simulink model "MultiUAV_DroneShow"  (R2026a)
settings: Solver=ode1  StopTime=74.3333  FixedStep=Ts_sim  MaxStep=0.01  AbsTol=1e-6
PreLoadFcn:
  | setupParams
values from neighbouring files (symbols this model uses):
  arm_duration = 2    [setupParams.m]
  gnss_deny_mask = false(N_uav, 1)    [setupParams.m]
  gnss_err_gain = sqrt(1 - gnss_err_pole^2)    [setupParams.m]
  gnss_err_pole = exp(-Ts_sim / gnss_err_tau)    [setupParams.m]
  gnss_err_seed = reshape(40000 + (1:(N_uav * 3)), N_uav, 3)    [setupParams.m]
  gps_accuracy_rtk_fix = 0.02    [setupParams.m]
  gps_lock_duration = 2    [setupParams.m]
  gravity = 9.81    [setupParams.m]
  hb_period_ticks = mavlink_hb_interval / Ts_sim    (= 100)    [setupParams.m]
  init_positions = init_positions(pad_of, :)    [planShow.m]    (also in setupParams.m = plan.init_positions)
  Kd_pos = repmat([Kd_xy Kd_xy Kd_z], N_uav, 1)    [setupParams.m]
  Kff_pos = Kd_pos    [setupParams.m]
  Kp_pos = repmat([Kp_xy Kp_xy Kp_z], N_uav, 1)    [setupParams.m]
  land_end_time = plan.land_end_time    [packShowUpload.m]    (also in planShow.m = show_flight_duration + land_duration; setupParams.m)
  land_speed = cfg.land_speed    [planShow.m]
  land_start_time = show_flight_duration    [planShow.m]    (also in setupParams.m = plan.land_start_time)
  land_total_duration = land_duration + land_settle    [planShow.m]    (also in setupParams.m = plan.land_total_duration)
  mav_sys_span = 250    [setupParams.m]
  N_uav = 20    [DroneShowExample.m]    (also in packShowUpload.m = cfg.N_uav; planShow.m = cfg.N_uav; setupParams.m = 10)
  num_waypoints = length(upload_times)    [packShowUpload.m]    (also in setupParams.m = pack.num_waypoints)
  rtcm_data_bytes = 180    [setupParams.m]
  rtcm_interval = 1.0    (= 1)    [setupParams.m]
  rtcm_payload_bytes = 4 * 4 * rtk_n_sat    [setupParams.m]
  rtcm_period_ticks = rtcm_interval / Ts_sim    (= 100)    [setupParams.m]
  rtk_amb_l1_base = 1000000 + mod(97 * (1:rtk_n_sat)', 1009)    [setupParams.m]
  rtk_amb_l1_rover = rtk_amb_l1_base + rtk_amb_l1    [setupParams.m]
  rtk_amb_l2_base = 1000000 + mod(89 * (1:rtk_n_sat)', 1009)    [setupParams.m]
  rtk_amb_l2_rover = rtk_amb_l2_base + rtk_amb_l2    [setupParams.m]
  rtk_base_lla = [42.3601, -71.0589, 10]    [setupParams.m]
  rtk_deny_mask = false(N_uav, 1)    [setupParams.m]
  rtk_f1 = 1575.42e6    (= 1575420000)    [setupParams.m]
  rtk_f2 = 1227.60e6    (= 1227600000)    [setupParams.m]
  rtk_fall_slew = -gps_accuracy_standard / reconverge_time    (= -0.3)    [setupParams.m]
  rtk_fix_thresh_l1 = 0.30    (= 0.3)    [setupParams.m]
  rtk_fix_thresh_wl = 0.25    [setupParams.m]
  rtk_inject_enable = double(~skip_preflight | rtk_deny_mask(:)')    [setupParams.m]
  rtk_lambda1 = rtk_c / rtk_f1    (= 0.190293672798)    [setupParams.m]
  rtk_lambda2 = rtk_c / rtk_f2    (= 0.244210213425)    [setupParams.m]
  rtk_lambda_wl = rtk_c / (rtk_f1 - rtk_f2)    (= 0.861918400322)    [setupParams.m]
  rtk_lock_dwell = 2.0    (= 2)    [setupParams.m]
  rtk_los = [cosd(rtk_el) .* sind(rtk_az), cosd(rtk_el) .* cosd(rtk_az), sind(rtk_el)]    [setupParams.m]
  rtk_mean_clk = zeros(2, 1)    [setupParams.m]
  rtk_mean_obs = zeros(2, rtk_n_sat)    [setupParams.m]
  rtk_n_sat = numel(rtk_az)    [setupParams.m]
  rtk_rough_range = pseudoranges(rtk_base_lla, rtk_sat_pos, 'RangeAccuracy', 0)    [setupParams.m]
  rtk_sat_pos = rtk_sat_pos_all(rtk_vis, :)    [setupParams.m]
  rtk_seedm_clk = 9101 + 8 * rtk_n_sat + (0:1)'    [setupParams.m]
  rtk_seedm_l1 = rtk_seedm_p2 + 2 * rtk_n_sat    [setupParams.m]
  rtk_seedm_l2 = rtk_seedm_l1 + 2 * rtk_n_sat    [setupParams.m]
  rtk_seedm_p1 = 9101 + reshape(0:2 * rtk_n_sat - 1, 2, rtk_n_sat)    [setupParams.m]
  rtk_seedm_p2 = rtk_seedm_p1 + 2 * rtk_n_sat    [setupParams.m]
  rtk_sigma_bp = [0, rtk_timeout, rtk_float_timeout]    [setupParams.m]
  rtk_sigma_table = sqrt(max(0, rtk_sigma_tiers.^2 - gps_accuracy_rtk_fix^2))    [setupParams.m]
  rtk_sigma_unfixed = 0.75    [setupParams.m]
  rtk_slip_thresh_l1 = 0.02    [setupParams.m]
  rtk_slip_thresh_wl = 0.10    (= 0.1)    [setupParams.m]
  rtk_status_l1 = 1    [setupParams.m]
  rtk_status_unfixed = 3    [setupParams.m]
  rtk_timeout = 2.5    [setupParams.m]
  rtk_var_clk = rtk_clock_sigma^2 * ones(2, 1)    [setupParams.m]
  rtk_var_l = [rtk_sigma_phase_base^2; rtk_sigma_phase_rover^2] * ones(1, rtk_n_sat)    [setupParams.m]
  rtk_var_p = [rtk_sigma_code_base^2;  rtk_sigma_code_rover^2 ] * ones(1, rtk_n_sat)    [setupParams.m]
  skip_preflight = traj_source == 1    [DroneShowExample.m]    (also in setupParams.m = false)
  st_period_ticks = mavlink_st_interval / Ts_sim    (= 100)    [setupParams.m]
  st_phase_ticks = st_period_ticks / 2    (= 50)    [setupParams.m]
  telemetry_tx_enable = double(~skip_preflight)    [setupParams.m]
  traj_upload_flat = zeros(N_uav*num_waypoints, 7)    [packShowUpload.m]    (also in setupParams.m = pack.traj_upload_flat)
  Ts_sim = cfg.Ts_sim    [packShowUpload.m]    (also in setupParams.m = 0.01)
  uav_loss_seed = 31000 + (1:N_uav)    [setupParams.m]
  uav_mass = 0.1    [setupParams.m]
  upload_duration = (total_packets + N_uav) * Ts_sim * 1.2    [packShowUpload.m]    (also in setupParams.m = pack.upload_duration)
  upload_rate_vec = [1 ./ upload_dt; 1 / upload_dt(end)]    [packShowUpload.m]    (also in setupParams.m = pack.upload_rate_vec)
  upload_request = traj_source == 2    [DroneShowExample.m]
undefined symbols (not defined in the file or in its folder): abort_request, DiscIntNeverNeededParam, doppler, loss_seed, packet_loss_rate, Payload, SystemID, uav_loss_rate
libraries: uavmavlinklib x22, hdlsllib x16, dspsigops x8, simulink x7, matrix_library x4, commchan3 x2, etargetslib x1, uavalgslib x1, sensorinslib x1, slpidlib x1, dspmathops x1, commrandsrc3 x1
(part 3 of 4)

== system MultiUAV_DroneShow/BaseStation/Transmitter/MissionItemTx/AddrSplit ==
  idx : Inport
  AddC1 : Sum  OutDataTypeStr=uint16
  AddS1 : Sum  OutDataTypeStr=uint16
  C_one : Constant  Value=uint16(1)  OutDataTypeStr=uint16
  C_span : Constant  Value=uint16(mav_sys_span)  OutDataTypeStr=uint16
  C_zero : Constant  Value=uint8(0)  OutDataTypeStr=uint8
  DTC_comp : DataTypeConversion  OutDataTypeStr=uint8
  DTC_sys : DataTypeConversion  OutDataTypeStr=uint8
  DivF : Product  Inputs=*/  OutDataTypeStr=uint16
  MaxIdx : MinMax  Function=max  Inputs=2  OutDataTypeStr=uint16
  MulS : Product  Inputs=**  OutDataTypeStr=uint16
  Sub1 : Sum  Inputs=+-  OutDataTypeStr=uint16
  SubS : Sum  Inputs=+-  OutDataTypeStr=uint16
  SwComp : Switch  Criteria=u2 > Threshold
  SwSys : Switch  Criteria=u2 > Threshold
  target_system : Outport
  target_component : Outport  Port=2
  wires:
  idx/1 -> MaxIdx/1, SwSys/2, SwComp/2
  C_one/1 -> MaxIdx/2, Sub1/2, AddS1/2, AddC1/2
  MaxIdx/1 -> Sub1/1
  Sub1/1 -> DivF/1, SubS/1
  C_span/1 -> DivF/2, MulS/2
  DivF/1 -> MulS/1, AddC1/1
  MulS/1 -> SubS/2
  SubS/1 -> AddS1/1
  AddS1/1 -> DTC_sys/1
  AddC1/1 -> DTC_comp/1
  DTC_sys/1 -> SwSys/1
  C_zero/1 -> SwSys/3, SwComp/3
  DTC_comp/1 -> SwComp/1
  SwSys/1 -> target_system/1
  SwComp/1 -> target_component/1

== system MultiUAV_DroneShow/BaseStation/Transmitter/RTCMTx/PackRTKDataBlk ==
  BaseObs : Inport
  BytePack : etargetslib/Byte Pack  datatypes={'single'}  byteAlign=1
  ConcatBytes : Concatenate
  DTC_single : DataTypeConversion  OutDataTypeStr=single
  PadZeros : Constant  Value=zeros(1,rtcm_data_bytes-rtcm_payload_bytes,'uint8')  OutDataTypeStr=uint8
  data : Outport
  wires:
  BytePack/1 -> ConcatBytes/1
  ConcatBytes/1 -> data/1
  PadZeros/1 -> ConcatBytes/2
  BaseObs/1 -> DTC_single/1
  DTC_single/1 -> BytePack/1

== system MultiUAV_DroneShow/DroneFleet/SetpointGenerator/PlannedTrajectory/OnboardTrajSource ==
  ShowTime : Inport
  BufferAsWpDroneXYZ : Reshape  OutputDimensionality=Customize  OutputDimensions=[num_waypoints, N_uav, 3]
  CatPosVelYaw : Concatenate  NumInputs=3  Mode=Multidimensional array  ConcatenateDimension=2
  FracOfDelta : Product
  GroundHold : Constant  Value=[init_positions'; zeros(4, N_uav)]
  IdxNext : Bias  Bias=2
  IdxThis : Bias  Bias=1
  NextWpPerDrone : Reshape  OutputDimensionality=Customize  OutputDimensions=[N_uav 3]
  OnboardPos : Sum  Inputs=|++
  OnboardVel : Product
  OnboardYaw : Constant  Value=zeros(N_uav,1)
  PickNextWp : Selector  NumberOfDimensions=3  IndexOptions=Index vector (port),Select all,Select all  Indices=1,1,1  OutputSizes=1,1,1
  PickThisWp : Selector  NumberOfDimensions=3  IndexOptions=Index vector (port),Select all,Select all  Indices=1,1,1  OutputSizes=1,1,1
  PickWpRate : Selector  InputPortWidth=num_waypoints  IndexOptions=Index vector (port)  Indices=1  OutputSizes=1
  PreShowGate : Switch  Criteria=u2 > Threshold
  ReadOnboardBuffer : DataStoreRead  DataStoreName=OnboardBuffer  IndexOptions=Index vector (dialog)  Indices=1  OutputSizes=1
  ThisWpPerDrone : Reshape  OutputDimensionality=Customize  OutputDimensions=[N_uav 3]
  ToSevenRows : Math  Operator=transpose
  WaypointLookup : PreLookup  BreakpointsData=upload_times
  WpDelta : Sum  Inputs=+-
  WpRateVec : Constant  Value=upload_rate_vec
  TrajMatrix : Outport
  wires:
  ShowTime/1 -> WaypointLookup/1, PreShowGate/2  "show_time"
  PickWpRate/1 -> OnboardVel/2
  WpRateVec/1 -> PickWpRate/1
  OnboardVel/1 -> CatPosVelYaw/2
  PreShowGate/1 -> TrajMatrix/1  "onboard_traj"
  GroundHold/1 -> PreShowGate/3
  ToSevenRows/1 -> PreShowGate/1
  CatPosVelYaw/1 -> ToSevenRows/1
  OnboardYaw/1 -> CatPosVelYaw/3
  OnboardPos/1 -> CatPosVelYaw/1  "onboard_pos"
  FracOfDelta/1 -> OnboardPos/2
  WpDelta/1 -> OnboardVel/1, FracOfDelta/2  "wp_delta"
  WaypointLookup/2 -> FracOfDelta/1
  ThisWpPerDrone/1 -> OnboardPos/1, WpDelta/2
  NextWpPerDrone/1 -> WpDelta/1
  PickNextWp/1 -> NextWpPerDrone/1
  PickThisWp/1 -> ThisWpPerDrone/1
  IdxNext/1 -> PickNextWp/2
  IdxThis/1 -> PickWpRate/2, PickThisWp/2
  BufferAsWpDroneXYZ/1 -> PickNextWp/1, PickThisWp/1
  ReadOnboardBuffer/1 -> BufferAsWpDroneXYZ/1  "onboard_wp"
  WaypointLookup/1 -> IdxNext/1, IdxThis/1

== system MultiUAV_DroneShow/DroneFleet/Transmitter/MissionAckEncoder/AckMsgGate ==
  In1 : Inport
  Enable : EnablePort
  AckType0 : Constant  Value=uint8(0)  OutDataTypeStr=uint8
  AddrSplit : Subsystem
  BlankMsg_MAck : uavmavlinklib/MAVLink Blank Message  dialectSource=Select from standard MAVLink dialects  dialect=common.xml  dialectCustom=common.xml  version=2  messageType=MISSION_ACK  SystemID=1  ComponentID=1  SampleTime=inf
  DTC_MAck : DataTypeConversion  OutDataTypeStr=uint8  SaturateOnIntegerOverflow=off  RndMeth=Floor
  Fill_MAck : BusAssignment  AssignedSignals=Payload.target_system,Payload.type,Payload.target_component
  Pad_MAck : dspsigops/Pad  padAlong=Rows  dimsToPad=1  valSrc=Specify via dialog  padVal=0  spec=Output size  padNumOutRowsSpecMethod=User-specified  numOutRows=1  padNumOutColsSpecMethod=User-specified  numOutCols=40  isVarDimsMode=off  padBeginning=0  padEnd=0  outSizeMode=User-specified  outSize=1  padSigAt=End  trunc_flag=None  roundingMode=Floor  overflowMode=off  truncOrWrapMode=Truncate  wrap_flag=None
  Ser_MAck : uavmavlinklib/MAVLink Serializer  dialectSource=Select from standard MAVLink dialects  dialect=common.xml  dialectCustom=common.xml  version=2  messageType=MISSION_ACK
  TermSerMAckLen : Terminator
  Out1 : Outport
  wires:
  Ser_MAck/1 -> Pad_MAck/1
  Ser_MAck/2 -> TermSerMAckLen/1
  BlankMsg_MAck/1 -> Fill_MAck/1
  Pad_MAck/1 -> DTC_MAck/1
  AckType0/1 -> Fill_MAck/3
  DTC_MAck/1 -> Out1/1
  Fill_MAck/1 -> Ser_MAck/1
  In1/1 -> AddrSplit/1(idx)
  AddrSplit/1(target_system) -> Fill_MAck/2
  AddrSplit/2(target_component) -> Fill_MAck/4

== system MultiUAV_DroneShow/DroneFleet/Transmitter/MissionRequestEncoder/ReqMsgGate ==
  In1 : Inport
  In2 : Inport  Port=2
  Enable : EnablePort
  AddrSplit : Subsystem
  BlankMsg_MReq : uavmavlinklib/MAVLink Blank Message  dialectSource=Select from standard MAVLink dialects  dialect=common.xml  dialectCustom=common.xml  version=2  messageType=MISSION_REQUEST_INT  SystemID=1  ComponentID=1  SampleTime=inf
  DTC_MReq : DataTypeConversion  OutDataTypeStr=uint8  SaturateOnIntegerOverflow=off  RndMeth=Floor
  Fill_MReq : BusAssignment  AssignedSignals=Payload.target_system,Payload.seq,Payload.target_component
  Pad_MReq : dspsigops/Pad  padAlong=Rows  dimsToPad=1  valSrc=Specify via dialog  padVal=0  spec=Output size  padNumOutRowsSpecMethod=User-specified  numOutRows=1  padNumOutColsSpecMethod=User-specified  numOutCols=40  isVarDimsMode=off  padBeginning=0  padEnd=0  outSizeMode=User-specified  outSize=1  padSigAt=End  trunc_flag=None  roundingMode=Floor  overflowMode=off  truncOrWrapMode=Truncate  wrap_flag=None
  Ser_MReq : uavmavlinklib/MAVLink Serializer  dialectSource=Select from standard MAVLink dialects  dialect=common.xml  dialectCustom=common.xml  version=2  messageType=MISSION_REQUEST_INT
  TermSerMReqLen : Terminator
  Out1 : Outport
  wires:
  BlankMsg_MReq/1 -> Fill_MReq/1
  Fill_MReq/1 -> Ser_MReq/1
  Ser_MReq/2 -> TermSerMReqLen/1
  Pad_MReq/1 -> DTC_MReq/1
  Ser_MReq/1 -> Pad_MReq/1
  In2/1 -> Fill_MReq/3
  DTC_MReq/1 -> Out1/1
  In1/1 -> AddrSplit/1(idx)
  AddrSplit/1(target_system) -> Fill_MReq/2
  AddrSplit/2(target_component) -> Fill_MReq/4

== system MultiUAV_DroneShow/RTKBase/ObservableSource/Simulated/ObservableGen ==
  RoverPos : Inport
  BreakLoop : UnitDelay  InitialCondition=[0;0;0]  SampleTime=rtcm_interval
  ClockOffset : RandomNumber  Mean=rtk_mean_clk  Variance=rtk_var_clk  Seed=rtk_seedm_clk  SampleTime=rtcm_interval
  HoldAtRTCMRate : ZeroOrderHold  SampleTime=rtcm_interval
  NoiseL1 : RandomNumber  Mean=rtk_mean_obs  Variance=rtk_var_l  Seed=rtk_seedm_l1  SampleTime=rtcm_interval
  NoiseL2 : RandomNumber  Mean=rtk_mean_obs  Variance=rtk_var_l  Seed=rtk_seedm_l2  SampleTime=rtcm_interval
  NoiseP1 : RandomNumber  Mean=rtk_mean_obs  Variance=rtk_var_p  Seed=rtk_seedm_p1  SampleTime=rtcm_interval
  NoiseP2 : RandomNumber  Mean=rtk_mean_obs  Variance=rtk_var_p  Seed=rtk_seedm_p2  SampleTime=rtcm_interval
  Observables : MATLAB Function  TreatAsAtomicUnit=on
  PickRover : Gain  Gain=[1 zeros(1,N_uav-1)]  Multiplication=Matrix(K*u)
  ToColumn : Reshape  OutputDimensionality=Customize  OutputDimensions=[3 1]
  P1 : Outport
  P2 : Outport  Port=2
  L1 : Outport  Port=3
  L2 : Outport  Port=4
  wires:
  Observables/3(L1) -> L1/1
  Observables/2(P2) -> P2/1
  NoiseL2/1 -> Observables/6(NoiseL2)
  NoiseL1/1 -> Observables/5(NoiseL1)
  NoiseP1/1 -> Observables/3(NoiseP1)
  HoldAtRTCMRate/1 -> BreakLoop/1
  Observables/1(P1) -> P1/1
  NoiseP2/1 -> Observables/4(NoiseP2)
  ToColumn/1 -> HoldAtRTCMRate/1
  Observables/4(L2) -> L2/1
  BreakLoop/1 -> Observables/1(Baseline)
  PickRover/1 -> ToColumn/1
  ClockOffset/1 -> Observables/2(Clock)
  RoverPos/1 -> PickRover/1

== system MultiUAV_DroneShow/DroneFleet/Transmitter/MissionAckEncoder/AckMsgGate/AddrSplit ==
  idx : Inport
  AddC1 : Sum  OutDataTypeStr=uint16
  AddS1 : Sum  OutDataTypeStr=uint16
  C_one : Constant  Value=uint16(1)  OutDataTypeStr=uint16
  C_span : Constant  Value=uint16(mav_sys_span)  OutDataTypeStr=uint16
  C_zero : Constant  Value=uint8(0)  OutDataTypeStr=uint8
  DTC_comp : DataTypeConversion  OutDataTypeStr=uint8
  DTC_sys : DataTypeConversion  OutDataTypeStr=uint8
  DivF : Product  Inputs=*/  OutDataTypeStr=uint16
  MaxIdx : MinMax  Function=max  Inputs=2  OutDataTypeStr=uint16
  MulS : Product  Inputs=**  OutDataTypeStr=uint16
  Sub1 : Sum  Inputs=+-  OutDataTypeStr=uint16
  SubS : Sum  Inputs=+-  OutDataTypeStr=uint16
  SwComp : Switch  Criteria=u2 > Threshold
  SwSys : Switch  Criteria=u2 > Threshold
  target_system : Outport
  target_component : Outport  Port=2
  wires:
  SwComp/1 -> target_component/1
  SwSys/1 -> target_system/1
  DTC_comp/1 -> SwComp/1
  C_zero/1 -> SwComp/3, SwSys/3
  DTC_sys/1 -> SwSys/1
  AddC1/1 -> DTC_comp/1
  AddS1/1 -> DTC_sys/1
  SubS/1 -> AddS1/1
  MulS/1 -> SubS/2
  DivF/1 -> AddC1/1, MulS/1
  C_span/1 -> MulS/2, DivF/2
  Sub1/1 -> SubS/1, DivF/1
  MaxIdx/1 -> Sub1/1
  C_one/1 -> AddC1/2, AddS1/2, Sub1/2, MaxIdx/2
  idx/1 -> SwComp/2, SwSys/2, MaxIdx/1

== system MultiUAV_DroneShow/DroneFleet/Transmitter/MissionRequestEncoder/ReqMsgGate/AddrSplit ==
  idx : Inport
  AddC1 : Sum  OutDataTypeStr=uint16
  AddS1 : Sum  OutDataTypeStr=uint16
  C_one : Constant  Value=uint16(1)  OutDataTypeStr=uint16
  C_span : Constant  Value=uint16(mav_sys_span)  OutDataTypeStr=uint16
  C_zero : Constant  Value=uint8(0)  OutDataTypeStr=uint8
  DTC_comp : DataTypeConversion  OutDataTypeStr=uint8
  DTC_sys : DataTypeConversion  OutDataTypeStr=uint8
  DivF : Product  Inputs=*/  OutDataTypeStr=uint16
  MaxIdx : MinMax  Function=max  Inputs=2  OutDataTypeStr=uint16
  MulS : Product  Inputs=**  OutDataTypeStr=uint16
  Sub1 : Sum  Inputs=+-  OutDataTypeStr=uint16
  SubS : Sum  Inputs=+-  OutDataTypeStr=uint16
  SwComp : Switch  Criteria=u2 > Threshold
  SwSys : Switch  Criteria=u2 > Threshold
  target_system : Outport
  target_component : Outport  Port=2
  wires:
  SwComp/1 -> target_component/1
  SwSys/1 -> target_system/1
  DTC_comp/1 -> SwComp/1
  C_zero/1 -> SwComp/3, SwSys/3
  DTC_sys/1 -> SwSys/1
  AddC1/1 -> DTC_comp/1
  AddS1/1 -> DTC_sys/1
  SubS/1 -> AddS1/1
  MulS/1 -> SubS/2
  DivF/1 -> AddC1/1, MulS/1
  C_span/1 -> MulS/2, DivF/2
  Sub1/1 -> SubS/1, DivF/1
  MaxIdx/1 -> Sub1/1
  C_one/1 -> AddC1/2, AddS1/2, Sub1/2, MaxIdx/2
  idx/1 -> SwComp/2, SwSys/2, MaxIdx/1

== stateflow chart MultiUAV_DroneShow/ShowSupervisor ==
  state IDLE
    entry:  NoFly=false;Phase=uint8(0); t_phase_start=t; UploadEnable=false; StartBroadcast=false; TimeBroadcastEnable=false; ShowTime=0; ClearFlags=false; LandNow=false;
  state UPLOADING
    entry: Phase=uint8(1); t_phase_start=t; UploadEnable=true; ClearFlags=true;
    during: ClearFlags=false;
    exit: UploadEnable=false;
  state UPLOAD_FAILED
    entry:
    % Latched: the operator must issue a NEW upload request to retry.
    Phase = uint8(6); UploadEnable = false; ClearFlags = false;
    prev_request = UploadRequest;
    during:
    prev_request = UploadRequest;
  state ARMED
    entry:  NoFly = ~RtkReady;Phase=uint8(2); t_phase_start=t;
    during: NoFly = ~RtkReady;
  state SHOW
    entry:  NoFly = false;Phase=uint8(3); t_phase_start=t; StartBroadcast=true; TimeBroadcastEnable=true;
    during: StartBroadcast=false; ShowTime=t-t_phase_start;
  state LANDING
    entry: Phase=uint8(5); LandNow=false;
    during:
    % Keep the show clock running: the descent is part of the uploaded plan, so the
    % reference only reaches the ground if ShowTime carries on past land_start_time.
    % t_phase_start is still SHOW's, so this is the same clock, not a new one.
    ShowTime = t - t_phase_start;
  state ABORT_LANDING
    entry:
    % Operator abort: the plan is abandoned and LandNowRef takes over the
    % position command, walking the fleet straight down from wherever it is.
    Phase = uint8(5); LandNow = true; TimeBroadcastEnable = false;
    t_phase_start = t;
  state LANDED
    entry:
    % Parked. Stopping the time broadcast here rather than on the way out of SHOW
    % is what lets the planned descent reach the drones on the MAVLink path.
    %
    % LandNow is deliberately left as it is. Whichever state got here has already set
    % it: false from LANDING, so the plan's own parked waypoints pass through; true
    % from ABORT_LANDING, so the fleet stays where the abort put it down instead of
    % being flown back up by a plan it abandoned.
    Phase = uint8(4); TimeBroadcastEnable = false;
  (default) -> IDLE
  IDLE -> UPLOADING [order 1] : [(t - t_phase_start) >= gps_lock_duration && UploadRequest]
  IDLE -> SHOW [order 2] : [(t - t_phase_start) >= gps_lock_duration && SkipPreflight]
  UPLOAD_FAILED -> UPLOADING : [UploadRequest && ~prev_request]
  UPLOADING -> UPLOAD_FAILED [order 3] : [AnyMissionError || (t - t_phase_start) >= (upload_duration + 5)]
  UPLOADING -> ABORT_LANDING [order 1] : [AbortRequest]
  UPLOADING -> ARMED [order 2] : [AllMissionAcked]
  ARMED -> ABORT_LANDING [order 1] : [AbortRequest]
  ARMED -> SHOW [order 2] : [(t - t_phase_start) >= arm_duration && RtkReady]
  SHOW -> ABORT_LANDING [order 1] : [AbortRequest]
  SHOW -> LANDING [order 2] : [ShowTime >= land_start_time]
  ABORT_LANDING -> LANDED : [(t - t_phase_start) >= land_total_duration]
  LANDING -> LANDED : [ShowTime >= land_end_time]
  data: AllMissionAcked input boolean; AnyMissionError input boolean; t input double; Phase output uint8; ShowTime output double; UploadEnable output boolean; StartBroadcast output boolean; TimeBroadcastEnable output boolean; t_phase_start local double; gps_lock_duration parameter double; upload_duration parameter double; arm_duration parameter double; UploadRequest input; ClearFlags output; prev_request local boolean size=[1 1] =0; SkipPreflight input boolean; AbortRequest input boolean; LandNow output boolean; land_start_time parameter double; land_total_duration parameter double; land_end_time parameter double; RtkReady input boolean; NoFly output boolean

== matlab function MultiUAV_DroneShow/RTKBase/RTKEngine/Cascade ==
  settings: updateMethod=DISCRETE  sampleTime=rtcm_interval
  data: P1 input; Baseline output; P2 input; L1 input; L2 input; LOS input; Valid input; Sigma output; Status output; Diag output; rtk_f1 parameter; rtk_f2 parameter; rtk_lambda_wl parameter; rtk_lambda1 parameter; rtk_fix_thresh_wl parameter; rtk_fix_thresh_l1 parameter; rtk_slip_thresh_wl parameter; rtk_slip_thresh_l1 parameter
function [Baseline, Sigma, Status, Diag] = rtkCascade(P1, P2, L1, L2, LOS, Valid, rtk_f1, rtk_f2, rtk_lambda_wl, rtk_lambda1, rtk_fix_thresh_wl, rtk_fix_thresh_l1, rtk_slip_thresh_wl, rtk_slip_thresh_l1)
%rtkCascade - double difference, Melbourne-Wubbena, integer fix. The RTK engine.
%
% This one block replaced the 123 that used to be RTKEngine: four subsystems of
% Product/Sum/Switch/UnitDelay chains implementing exactly the arithmetic below. Arm 10 of
% tests/checkRTKEngine runs this block and tests/rtkReference.m -- an independently written
% MATLAB implementation of the same cascade -- on the SAME injected observables and demands
% agreement to 1e-9 on the baseline, the sigma AND the fix status, including the epochs where a
% wrong integer set is refused and re-resolved.
%
% Why one MATLAB Function block rather than blocks. The usual argument for blocks is that the
% algorithm becomes visible; here it did the opposite. This is dense linear algebra over a
% differencing operator with per-satellite latches layered on top, so in blocks the algebra
% lived inside Product blocks whose meaning was a matrix name, and the state was spread over
% seven UnitDelays with the latch conditions as Switch trees. And the usual toolbox argument
% does not apply either: not one of the 123 blocks was a toolbox block. They were all
% primitives.
%
% THE INTERFACE: UNDIFFERENCED OBSERVABLES, ONE ROW PER RECEIVER. P1/P2/L1/L2 are each
% 2-by-nSat -- the BASE row first, then the ROVER row -- carrying the raw code and phase each
% receiver measured, in metres. The between-receiver difference is formed HERE, in step 1
% below, not by whatever supplies the measurements.
%
% That boundary is the whole point of the block. A real base station and a real rover each
% report their own raw observables and nothing else: no receiver differences anything against
% a peer it has never heard of. So an interface that demanded the single difference would be
% asking its source for a quantity that cannot be measured, only constructed -- and would
% therefore need a different source for simulation than for real measurements. Undifferenced
% rows mean ObservableGen and a RINEX file enter by the same door, and arm 15 measures the
% only numerical cost of that (8.8e-9 m, 4.0e-6 of the phase noise, which is 2.4x eps at the
% raw magnitude: base and rover agree to a part in 6774, so the subtraction itself is exact and
% all that is left is the rounding of representing a raw observable at all).
%
% COLUMNS ARE SATELLITE SLOTS, AND Valid SAYS WHICH ARE OBSERVED. This is the rest of the
% contract, and everything below depends on it: column s of P1/P2/L1/L2 -- and row s of LOS and
% Valid -- refers to the SAME satellite on every epoch, and Valid(s) says whether that
% satellite was observed this epoch. Whatever supplies the measurements owns the PRN-to-slot
% map; the engine never sees a PRN. Get this wrong -- compact the slots each epoch so that slot
% 3 is "the third satellite currently up" -- and the engine silently attributes one satellite's
% accumulated ambiguity to another. Nothing errors; the fix just quietly resolves to the wrong
% integers.
%
% The alternative was to keep the observables packed and pass a satellite-count. That cannot
% work, because the state below is per satellite and has to survive a satellite disappearing
% from the middle of the list.
%
% WHY SATELLITES HAVE TO BE ABLE TO RISE AND SET. Until this change the engine assumed a fixed
% set: the accumulator and the held integers were indexed by DOUBLE-DIFFERENCE ROW, and a row
% meant "the k-th non-pivot satellite". In simulation that is stable because the constellation
% is frozen. Point the same engine at a real observation file and it is not: the one hour of
% GPS observations shipped with MATLAB has satellite arcs of 120, 120, 120, 120, 120, 97, 120,
% 120, 120, 81 and 61 epochs, so satellites genuinely rise and set INSIDE any subportion long
% enough to fix. With row-indexed state, a satellite setting shifts every row after it and the
% engine carries on using the accumulated ambiguity of a satellite that is no longer there.
%
% GEOMETRY IS AN INPUT, NOT A PARAMETER. This block used to take rtk_D, rtk_A, rtk_G and
% rtk_sigma_gain as parameters -- four matrices setupParams built once from the constellation
% visible over the base station at rtk_epoch. That is exact in simulation for a reason that
% does not survive contact with a real receiver: the SAME frozen constellation both generated
% the observables and solved them, so the satellite motion cancelled out of the estimate
% identically. Feed in observables that carry true moving geometry and the frozen gain costs
%
%     +  38 s  (one show)   0.312 deg of line-of-sight change ->  0.61 m of baseline error
%     + 124 s               1.019 deg                         ->  1.97 m
%     + 600 s               the visible set has churned; the rows are different satellites
%
% None of that announces itself: it degrades quietly and then breaks structurally the first
% time a satellite rises or sets. So the four matrices are now rebuilt every epoch from LOS.
%
% LOS is ENU rather than ECEF satellite positions deliberately. The engine is ENU end to end --
% the baseline it reports is ENU -- so putting the coordinate rotation in here would make the
% estimator responsible for a frame conversion that belongs to whatever is supplying the
% measurements. A real source has satellite positions in ECEF (gnssmeasurements returns them
% in its SatellitePosition column); converting them to unit line-of-sight vectors at the base
% station is the source's job, and elevation -- needed only to pick the pivot -- comes back out
% of LOS as asind(LOS(:,3)) at no cost.
%
% THE CASCADE -- tests/rtkReference.m carries the long form of why each step is what it is.
%   1. Single difference between RECEIVERS, rover minus base. Cancels everything that belongs
%      to the satellite and the epoch rather than to a receiver: the satellite clock bias, the
%      Earth-rotation correction, and the bulk of the atmosphere over a short baseline. Arm 12
%      measures the first two cancelling by a factor of 26246.
%   2. Double difference between SATELLITES. Differencing again against the pivot satellite
%      cancels both receiver clocks EXACTLY. That is the step position-domain DGPS has no
%      analogue of, and arm 1 is the proof: 900 m of receiver clock moves the reported baseline
%      by 6e-13 m, while the same data undifferenced is 1162 m out. Note that arm 1 now tests
%      THIS BLOCK -- the two clocks arrive independently on the two rows, so it is step 1 and
%      step 2 together that remove them, where before the source handed over the difference.
%   3. Melbourne-Wubbena. Wide-lane phase minus narrow-lane code is free of BOTH geometry and
%      ionosphere, so its ambiguity can be averaged straight down out of the code noise with
%      no position estimate at all.
%   4. Wide-lane fix. Round the average and accept it when every element is within
%      rtk_fix_thresh_wl of an integer. 0.862 m of wavelength makes this the easy fix.
%   5. L1 fix, conditioned on the wide-lane baseline. With a centimetre baseline in hand the
%      float L1 ambiguity is good to a few hundredths of a cycle and rounds on sight; 0.190 m
%      of wavelength then makes this the accurate one.
%
% Both held integer sets are re-validated on EVERY epoch, not only when they are accepted. A
% wrong set is self-consistent -- the fit closes around a baseline metres out and the residual
% comes back at the phase noise floor -- so no accuracy check downstream can tell it is wrong.
% Arm 9 turns the wide-lane validation off and the same seeds then hold 0.3 m of error for the
% whole show without ever once reporting worse than a carrier-phase fix.
%
% Diag exists for the tests, not for the show:
%   [wide-lane latch engaged; the wide-lane fit accepted it; L1 latch engaged; L1 fit accepted]
% A rejection cannot be seen in Status. The latch and its validation happen in the SAME epoch,
% so a bad set is thrown out before it is ever reported and Status simply stays at 3 -- which
% means counting "status got worse" finds nothing and passes arm 10 while proving nothing.
%#codegen

ns = size(LOS, 1);
vis = Valid(:) > 0.5;

% ---- 1. single difference between receivers, rover minus base ------------------------------
% The first line of the cascade, and the whole reason the interface is undifferenced. Row 2 is
% the rover, row 1 is the base; the sign convention is rover MINUS base, so a positive single
% difference means the rover is further from that satellite, and the baseline that comes out is
% the rover's position relative to the base. Reverse it and the engine returns a mirrored
% baseline that still fixes integers perfectly -- there is nothing self-inconsistent about the
% wrong sign, which is why the shape and order are checked at both sources rather than assumed.
%
% Everything downstream works on these O(100 m) differences, so the raw 2.3e7 m magnitudes exist
% only on these four input rows. That is what keeps arm 10 bit-exact against the reference: both
% implementations perform the identical elementwise subtraction on identical inputs, and no raw
% value survives past this point.
%
% Slots that are not observed are differenced anyway rather than guarded. They contribute
% nothing -- ddGeom gives them a zero row -- but the arithmetic has to stay finite, because a
% zero row of D still multiplies the whole vector and 0 * NaN is NaN. So the contract is that an
% unobserved slot carries a finite value, not that it carries a meaningful one.
p1 = (P1(2, :) - P1(1, :))';
p2 = (P2(2, :) - P2(1, :))';
l1 = (L1(2, :) - L1(1, :))';
l2 = (L2(2, :) - L2(1, :))';

% ---- state, one entry per SATELLITE SLOT ---------------------------------------------------
% mwAcc/mwN are the Melbourne-Wubbena arc for each satellite and are deliberately NEVER reset
% while the satellite stays up, not even when a held set is dropped: they keep averaging while
% the latch is clear, so a retry is better informed than the attempt that just failed and
% converges instead of starting over.
%
% mwN is per slot rather than a single epoch counter because satellites now have different arc
% lengths -- a satellite that rose 20 epochs into the run has averaged 20 epochs of noise down,
% not 200, and dividing its sum by the run length would report a fraction of the ambiguity.
persistent mwAcc mwN nWL heldWL nL1 heldL1 pivHeld
if isempty(mwN)
    mwAcc  = zeros(ns, 1);
    mwN    = zeros(ns, 1);
    nWL    = zeros(ns, 1);
    nL1    = zeros(ns, 1);
    heldWL = false(ns, 1);
    heldL1 = false(ns, 1);
    pivHeld = 0;
end

% ---- a slot that lost its satellite loses its arc ------------------------------------------
% Not merely "stop using it": clear it. A satellite that sets and rises again half an hour
% later has a NEW cycle ambiguity -- the receiver lost lock, so the integer count restarts --
% and carrying the old arc across the gap would latch a stale integer with high confidence,
% because mwN would say it had been averaged for hundreds of epochs.
for s = 1:ns
    if ~vis(s)
        mwAcc(s)  = 0;
        mwN(s)    = 0;
        nWL(s)    = 0;
        nL1(s)    = 0;
        heldWL(s) = false;
        heldL1(s) = false;
    end
end

% ---- pivot selection, with hysteresis while a fix is held ----------------------------------
% Highest satellite, because the pivot's own noise enters every single one of the differences,
% so it should be the least noisy one available. LOS(:,3) is sin(elevation), monotonic in
% elevation, so its argmax IS the highest satellite and no trigonometry is needed.
%
% But once integers are held they are held RELATIVE TO A PIVOT, so changing the pivot changes
% what every one of them means. Two satellites swapping places in elevation is common and
% costs nothing physically, and re-resolving the whole set every time that happened would
% throw away minutes of averaging for no reason. So while a fix is held the pivot stays put.
pivBest = 0;
bestEl  = -2;
for s = 1:ns
    if vis(s) && LOS(s, 3) > bestEl
        bestEl  = LOS(s, 3);
        pivBest = s;
    end
end
if any(heldWL) && pivHeld > 0 && vis(pivHeld)
    piv = pivHeld;
else
    piv = pivBest;
end

% The pivot had to move while integers were held, which happens only when the old pivot set.
% If the new pivot is itself in the held set the whole set can be re-referenced to it EXACTLY,
% because a double-difference ambiguity is a difference of two single-difference integers:
% N(s,new) = N(s,old) - N(new,old). That is integer arithmetic, so nothing is lost. If the new
% pivot is NOT held -- it just rose, say -- there is no such relation and the honest thing is
% to drop the fix and re-resolve, which the accumulators above make cheap.
if any(heldWL) && piv > 0 && piv ~= pivHeld
    if heldWL(piv)
        offWL = nWL(piv);
        offL1 = nL1(piv);
        for s = 1:ns
            if heldWL(s)
                nWL(s) = nWL(s) - offWL;
            end
            if heldL1(s)
                nL1(s) = nL1(s) - offL1;
            end
        end
        % The pivot has no ambiguity of its own: its double difference is identically zero.
        heldWL(piv) = false;
        heldL1(piv) = false;
        nWL(piv)    = 0;
        nL1(piv)    = 0;
    else
        for s = 1:ns
            heldWL(s) = false;
            heldL1(s) = false;
        end
    end
end
pivHeld = piv;

% ---- Melbourne-Wubbena, accumulated per satellite in SINGLE difference ---------------------
% Per satellite, NOT per double difference, and that is the change that lets the constellation
% move. The reason it is allowed: Melbourne-Wubbena is wide-lane phase minus narrow-lane code,
% and the receiver clock enters phase and code with the SAME coefficient (both are ranges in
% metres), so it cancels in the combination -- (f1*L1 - f2*L2)/(f1-f2) and (f1*P1 + f2*P2)/
% (f1+f2) each carry the clock with coefficient exactly 1. So the per-satellite MW is already
% clock-free without any differencing, and what is left is the ambiguity plus noise.
%
% That makes the accumulator PIVOT-INDEPENDENT. The double difference is recovered at the point
% of use as mwBar(s) - mwBar(piv), so when the pivot changes nothing has to be re-referenced
% and when a satellite rises it starts its own arc without disturbing anyone else's. Had the
% accumulator stayed in double-difference form, every pivot change would have needed a
% re-reference that is only exact when the two satellites have averaged the same epochs.
%
% One assumption is doing work here, and it is worth naming because a real receiver tests it:
% what survives in the single difference is the ambiguity plus a hardware bias (the phase and
% code delays of the two receivers). That bias has to be satellite-INDEPENDENT and constant for
% the difference against the pivot to remove it. It is, to well within a wide-lane cycle, which
% is why MW ambiguity resolution works on real data at all.
for s = 1:ns
    if vis(s)
        phiWLs   = (rtk_f1 * l1(s) - rtk_f2 * l2(s)) / (rtk_f1 - rtk_f2);
        pNLs     = (rtk_f1 * p1(s) + rtk_f2 * p2(s)) / (rtk_f1 + rtk_f2);
        mwAcc(s) = mwAcc(s) + (phiWLs - pNLs) / rtk_lambda_wl;
        mwN(s)   = mwN(s) + 1;
    end
end

mwBar = zeros(ns, 1);
for s = 1:ns
    if mwN(s) > 0
        mwBar(s) = mwAcc(s) / mwN(s);
    end
end

% ---- code-only baseline: the fallback, and the whole of what DGPS could ever manage --------
% Over EVERY valid satellite, not just the ones with resolved integers. The code solution is
% what the engine falls back to, so restricting it to the fixed subset would make the fallback
% worse the moment a satellite rose.
useCode = vis;
if piv > 0
    useCode(piv) = false;
end
[Dc, Ac, Gc, gainC, ~, okC] = ddGeom(useCode, piv, LOS, ns);

Baseline = zeros(3, 1);
% A satellite count below four is not a small error, it is no solution: three double
% differences fit three unknowns exactly, so the residual is identically zero and the
% validation below cannot fail. So report a sigma far outside every tier rtk_sigma_tiers
% defines, and let every consumer classify the epoch as unusable, which is what it is. Zero
% would read downstream as a perfect fix -- the exact inversion of the truth -- and Inf would
% put a non-finite value through a rate transition and a display. The show never reaches here:
% the simulated source is always 8 for 8.
Sigma  = 1e3;
Status = 3;
wlOK = false;  l1Held = false;  l1OK = false;   % the "not reached" values, so a stage that is
                                                % skipped reports skipped rather than accepted

if okC
    ddP1    = Dc * p1;
    bCode   = Gc * ddP1;
    resCode = ddP1 - Ac * bCode;
    Baseline = bCode;
    Sigma    = gainC * norm(resCode);
end

% ---- wide-lane latch ----------------------------------------------------------------------
% The double difference of the averaged MW, formed only now, from two pivot-independent arcs.
wlHeld = any(heldWL);
if piv > 0 && mwN(piv) > 0
    if ~wlHeld
        % All or nothing over the currently visible non-pivot satellites, which is what the
        % fixed-constellation version did and what arms 10 and 11 measure. Accepting on a
        % single epoch is only safe because of the validation below: a running mean can pass
        % the distance-to-integer test transiently while drifting past the WRONG integer, and
        % the defence against that is detection, not a longer wait here.
        allNear = true;
        nCand   = 0;
        for s = 1:ns
            if vis(s) && s ~= piv
                nCand = nCand + 1;
                f = mwBar(s) - mwBar(piv);
                if abs(f - round(f)) >= rtk_fix_thresh_wl
                    allNear = false;
                end
            end
        end
        if allNear && nCand >= 4
            for s = 1:ns
                if vis(s) && s ~= piv
                    nWL(s)    = round(mwBar(s) - mwBar(piv));
                    heldWL(s) = true;
                end
            end
        end
    else
        % A fix is already held and a satellite has since risen. Let it join on its own
        % merits rather than making the whole set wait for it -- and rather than excluding it
        % for the rest of the show, which is what a single all-or-nothing latch would do. Its
        % own arc is what is tested, so a satellite that just appeared cannot join until it
        % has averaged enough epochs to sit within the threshold, exactly like the first
        % latch. Note this branch cannot fire on a fixed constellation, so it costs arms 10
        % and 11 nothing.
        for s = 1:ns
            if vis(s) && s ~= piv && ~heldWL(s) && mwN(s) > 0
                f = mwBar(s) - mwBar(piv);
                if abs(f - round(f)) < rtk_fix_thresh_wl
                    nWL(s)    = round(f);
                    heldWL(s) = true;
                end
            end
        end
    end
end

% ---- wide-lane fit, re-validated on every epoch -------------------------------------------
bWL   = zeros(3, 1);
sigWL = 0;
AWL   = zeros(ns, 3);
Dw    = zeros(ns, ns);      % pre-declared: the L1 section reads it under a guard that implies
                            % it was assigned, but Coder's data flow analysis does not know that
wlHeld = any(heldWL);
if wlHeld
    useWL = heldWL & vis;
    [Dw, AWL, Gw, gainW, nW, okW] = ddGeom(useWL, piv, LOS, ns);
    if okW
        % Wide-lane phase with its integer removed is an unambiguous range observable at
        % ~13 mm of noise instead of 335 mm. Hence centimetres from carrier phase alone.
        phiWL = (rtk_f1 * (Dw * l1) - rtk_f2 * (Dw * l2)) / (rtk_f1 - rtk_f2);
        obsWL = phiWL - rtk_lambda_wl * (useWL .* nWL);
        bWL   = Gw * obsWL;
        resWL = obsWL - AWL * bWL;
        sigWL = gainW * norm(resWL);
        wlOK  = norm(resWL) / sqrt(max(1, nW - 3)) <= rtk_slip_thresh_wl;
    else
        % Too few satellites carry a resolved integer to fit anything, so the held set cannot
        % be validated and must not be reported.
        wlOK = false;
    end
    if ~wlOK
        for s = 1:ns
            heldWL(s) = false;
            heldL1(s) = false;                  % L1 is conditioned on the wide lane
        end
    end
end

% ---- L1 fix, conditioned on a baseline already good to centimetres ------------------------
bL1   = zeros(3, 1);
sigL1 = 0;
if wlHeld && wlOK
    ddL1w = AWL * bWL;                          % predicted, on the wide-lane geometry
    ddL1  = Dw * l1;                            % same rows, same subset, no pivot special case
    % All or nothing on the FIRST latch, exactly like the wide lane. Per satellite looked
    % defensible here on the argument that L1 has no accumulator -- each ambiguity is read off
    % a single epoch against a baseline that is ALREADY good to centimetres, so one marginal
    % satellite should not hold up the others. But that premise only holds when the WIDE-LANE
    % set is right. When it is wrong, a per-satellite latch finds whichever subset happens to
    % round cleanly around a baseline a metre out, that subset then fits itself, and the epoch
    % is reported as L1-fixed. Arm 9 measured it: with wide-lane validation disabled, two of
    % the five bad-latch seeds latched 6 of 7 slots and claimed millimetres at 0.31 m and
    % 0.84 m of real error. Requiring every wide-lane satellite to agree is what denies a wrong
    % baseline a consistent subset to hide in.
    if ~any(heldL1)
        allNear1 = true;
        for s = 1:ns
            if heldWL(s)
                n1hat = (ddL1(s) - ddL1w(s)) / rtk_lambda1;
                if abs(n1hat - round(n1hat)) >= rtk_fix_thresh_l1
                    allNear1 = false;
                end
            end
        end
        if allNear1
            for s = 1:ns
                if heldWL(s)
                    nL1(s)    = round((ddL1(s) - ddL1w(s)) / rtk_lambda1);
                    heldL1(s) = true;
                end
            end
        end
    else
        % An L1 fix is up and has passed its own validation, so the baseline really is good
        % and a satellite that rose late can join on its own merits rather than being shut out
        % for the rest of the show.
        for s = 1:ns
            if heldWL(s) && ~heldL1(s)
                n1hat = (ddL1(s) - ddL1w(s)) / rtk_lambda1;
                if abs(n1hat - round(n1hat)) < rtk_fix_thresh_l1
                    nL1(s)    = round(n1hat);
                    heldL1(s) = true;
                end
            end
        end
    end
    l1Held = any(heldL1);
    if l1Held
        useL1 = heldL1 & vis;
        [Dl, Al, Gl, gainL, nL, okL] = ddGeom(useL1, piv, LOS, ns);
        if okL
            obsL1 = (Dl * l1) - rtk_lambda1 * (useL1 .* nL1);
            bL1   = Gl * obsL1;
            resL1 = obsL1 - Al * bL1;
            sigL1 = gainL * norm(resL1);
            l1OK  = norm(resL1) / sqrt(max(1, nL - 3)) <= rtk_slip_thresh_l1;
        else
            l1OK = false;
        end
        if ~l1OK
            for s = 1:ns
                heldL1(s) = false;
            end
        end
    end
end

% ---- report the best state that survived validation this epoch ----------------------------
% A held L1 set whose fit was just refused falls back to the wide lane, not to code: the wide
% lane is still valid, and dropping all the way to a metre would be reporting worse than the
% engine knows.
if l1Held && l1OK
    Baseline = bL1;
    Sigma    = sigL1;
    Status   = 1;
elseif wlHeld && wlOK
    Baseline = bWL;
    Sigma    = sigWL;
    Status   = 2;
end

Diag = [double(wlHeld); double(wlOK); double(l1Held); double(l1OK)];
end


% -------------------------------------------------------------------------------------------
function [D, A, G, gain, nUse, ok] = ddGeom(use, piv, LOS, ns)
%ddGeom - differencing operator, design matrix, least-squares gain and sigma gain for one
% subset of satellites, all referenced to satellite `piv`.
%
% Called up to three times per epoch with three different subsets, because the code solution
% uses every visible satellite while the two fixed solutions use only those carrying a resolved
% integer. Sharing one geometry between them would either restrict the fallback to the fixed
% subset or include unresolved satellites in the fixed fit; both are wrong, and the matrices are
% tens of doubles, so recomputing is the cheap option.
%
% ROWS ARE SATELLITE SLOTS. Row s is the double difference of satellite s against the pivot, and
% is identically ZERO for a satellite that is not in `use`. That padding is not a compromise: a
% zero row of D contributes a zero row and column to Q = D*D', and a zero row of A gives a zero
% column of G, so every trace and every product below is EXACTLY the value the packed nUse-by-3
% form would give. Keeping the rows in slot order is what makes the per-satellite state above
% indexable at all -- pack the rows and row 4 means a different satellite on the next epoch.
%
% piv == 0 means no pivot: rows are single differences and Q comes out as I rather than
% I + ones. tests/rtkReference uses that to run its undifferenced control arm through the same
% code path, which is also the arm that shows the receiver clocks not cancelling.

D = zeros(ns, ns);
A = zeros(ns, 3);
nUse = 0;
for s = 1:ns
    if use(s) && s ~= piv
        D(s, s) = 1;
        A(s, :) = -LOS(s, :);
        if piv > 0
            D(s, piv) = D(s, piv) - 1;
            A(s, :)   = A(s, :) + LOS(piv, :);
        end
        nUse = nUse + 1;
    end
end

G    = zeros(3, ns);
gain = 0;
% Four, not three. Three double differences determine three unknowns exactly, so the residual
% is identically zero, the sigma gain is 0/0, and -- worse than either -- the every-epoch
% re-validation that arm 9 shows is load-bearing can never fail. An engine that cannot detect a
% wrong integer set must not report a fix.
ok = nUse >= 4;
if ~ok
    return
end

G = (A' * A) \ A';

% Live sigma as a single gain on the residual norm. Q = D*D' is I + ones over the used rows,
% not I, because every double difference contains the pivot satellite and they are therefore
% CORRELATED -- treating them as independent makes the reported sigma 1.42x optimistic, which is
% an error in the one direction that matters. The measurement variance cancels between the
% position covariance and the expected residual, so this ratio is pure geometry.
Q    = D * D';
M    = eye(ns) - A * G;
gain = sqrt(trace(G * Q * G') / trace(M * Q));
end
